simulink model "PowertrainV4"  (R2020b)
settings: Solver=VariableStepAuto  StartTime=0.0  StopTime=3000  MaxStep=0.06  RelTol=1e-3
values from neighbouring files (symbols this model uses):
  b = b +0.0001    (= 0.000245823376094)    [MotorSpecsForSimscape.m]
  F_drag = 0.5*1.2*0.089*0.42    (= 0.022428)    [MotorSpecsForSimscape.m]
  F_roll = 120 * 9.81 * 0.005    (= 5.886)    [MotorSpecsForSimscape.m]
  gearR = 46/11    (= 4.18181818182)    [MotorSpecsForSimscape.m]
  K = 0.0385    [MotorSpecsForSimscape.m]
  R = 0.103    [MotorSpecsForSimscape.m]
  Rs = 0.4    [MotorSpecsForSimscape.m]
  startup_t = 50    [MotorSpecsForSimscape.m]
  V_control = 24    [MotorSpecsForSimscape.m]
libraries: fl_lib x22, nesl_utility x11, sdl_lib x4, ee_lib x2
settings Model: Creator=Tom  LastModifiedBy=Tom
settings SolverCC: InitialStep=0.025

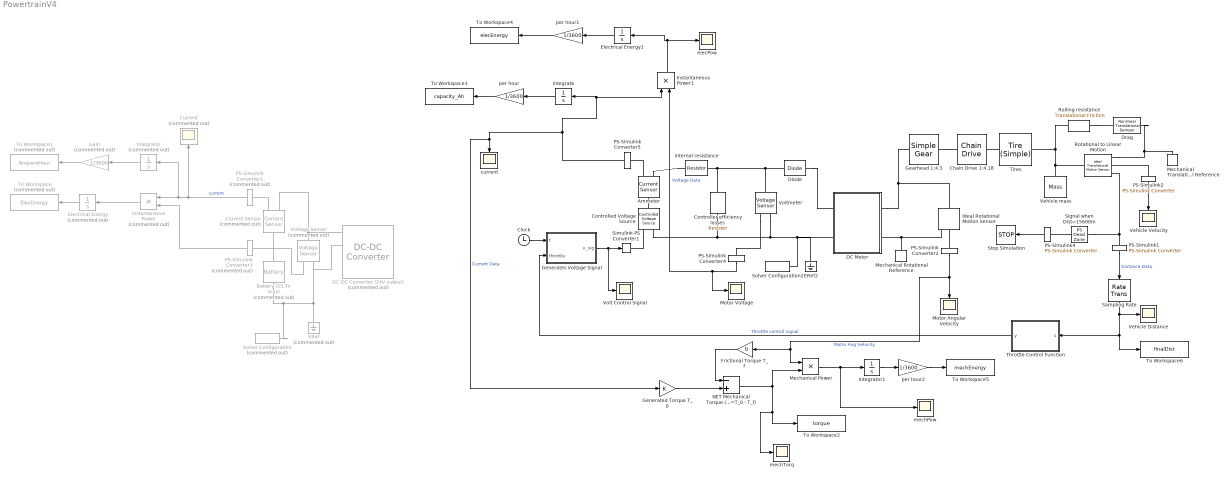
== system PowertrainV4 ==
  " Controlled Voltage Source" : fl_lib/Electrical/Electrical Sources/Controlled Voltage Source
  Ammeter : fl_lib/Electrical/Electrical Sensors/Current Sensor
  Battery (53.3V max) : ee_lib/Sources/Battery  Commented=on  Vnom=V0 V  prm_dir=1  R1_dis=2 Ohm  R1_ch=2 Ohm  R1=Rs Ohm  prm_AH=2  AH=AH0 hr*A  V1=V1 V  AH1=AH1 hr*A  prm_R2=1  R2=2000 Ohm  prm_dyn=1  Rp1=0.005 Ohm  tau1=30 s  Rp2=0.005 Ohm  tau2=30 s  Rp3=0.005 Ohm  tau3=30 s  Rp4=0.005 Ohm  tau4=30 s  Rp5=0.005 Ohm  tau5=30 s  prm_fade=1  N_fade=100  AH_fade=45 hr*A  R1_fade=2.02 Ohm  R1_ch_fade=2.02 Ohm  V1_fade=10.35 V  i_specify=off  i_priority=None  i=0 A  i_nominal_specify=off  i_nominal_unit=A  i_nominal_value=1  v_specify=off  v_priority=None  v=0 V  v_nominal_specify=off  v_nominal_unit=V  v_nominal_value=1  charge_specify=on  charge_priority=High  charge=AH0 hr*A  charge_nominal_specify=off  charge_nominal_unit=hr*A  charge_nominal_value=1  num_cycles_specify=off  num_cycles_priority=High  num_cycles=0  num_cycles_nominal_specify=off  num_cycles_nominal_unit=1  num_cycles_nominal_value=1  thermal_mass=30000 J/K  Tmeas=298.15 K  Vnom_T2=12 V  R1_T2=2.2 Ohm  R1_T2_dis=2.2 Ohm  R1_T2_ch=2.2 Ohm  V1_T2=11.4 V  R2_T2=2200 Ohm  Rp1_T2=0.005 Ohm  tau1_T2=30 s  Rp2_T2=0.005 Ohm  tau2_T2=30 s  Rp3_T2=0.005 Ohm  tau3_T2=30 s  Rp4_T2=0.005 Ohm  tau4_T2=30 s  Rp5_T2=0.005 Ohm  tau5_T2=30 s  Tmeas2=273.15 K  temperature_specify=off  temperature_priority=High  temperature=298.15 K  temperature_nominal_specify=off  temperature_nominal_unit=K  temperature_nominal_value=1
  Chain Drive 1:4.18 : sdl_lib/Couplings & Drives/Chain Drive  chain_model=sdl.enum.chain_model.ideal  radius_a=20 mm  radius_b=20*gearR mm  slack=50 mm  k_chain=1e5 N/m  mu_visc_chain=5 N/(m/s)  mu_visc_a=0 N*m/(rad/s)  mu_visc_b=0 N*m/(rad/s)  breakable=sdl.enum.max_tension.off  F_max=1e6 N  x_specify=off  x_priority=High  x=0 mm  x_nominal_specify=off  x_nominal_unit=mm  x_nominal_value=1
      settings: SourceProductBaseCode=LD  InternalSimscapePortConfiguration="{\"Bottom\":[],\"Left\":[{\"id\":\"A\",\"label\":\"A\",\"type\":\"foundation.mechanical.rotational.rotational\"}],\"Right\":[{\"id\":\"B\",\"label\":\"B\",\"type\":\"foundation.mechanical.rotational.rotational\"}],\"Top\":[]}"
  "Clock " : Clock
  Controller efficiency losses : fl_lib/Electrical/Electrical Elements/Resistor  R=30 Ohm  i_specify=off  i_priority=None  i=0 A  i_nominal_specify=off  i_nominal_unit=A  i_nominal_value=1  v_specify=off  v_priority=None  v=0 V  v_nominal_specify=off  v_nominal_unit=V  v_nominal_value=1
  Current : Scope  Commented=on
  Current Sensor : fl_lib/Electrical/Electrical Sensors/Current Sensor  Commented=on
  DC Motor : Subsystem
  "DC-DC Converter (24V output) " : ee_lib/Semiconductors & Converters/Converters/DC-DC Converter  Commented=on  Vref_option=ee.enum.converters.voltageref.external  v_ref=V_control V  P_rated=200 W  droop_param=1  droop=0.1 V/A  droop_percent=2  reversible=0  efficiency=0.9  P_fixed=1 W  model_dynamics=0  tau=0.02 s  v_ini=10 V  G_diode=1e-8 1/Ohm  i1_max=300 A  fault_condition=1  fault_threshold=0.5  thermal_mass=100 J/K  initial_temperature=298.15 K
      settings: SourceProductBaseCode=PS  InternalSimscapePortConfiguration="{\"Bottom\":[],\"Left\":[{\"id\":\"p1\",\"label\":\"1+\",\"type\":\"foundation.electrical.electrical\"},{\"id\":\"n1\",\"label\":\"1-\",\"type\":\"foundation.electrical.electrical\"},{\"id\":\"Vref\",\"label\":\"Vref\",\"type\":\"input\"},{\"id\":\"F\",\"label\":\"F\",\"type\":\"input\"}],\"Right\":[{\"id\":\"p2\",\"label\":\"2+\",\"type\":\"foundation.electrical.electrical\"},{\"id\":\"n2\",\"label\":\"2-\",\"type\":\"foundation.electrical.electrical\"}],\"Top\":[]}"
  Diode : fl_lib/Electrical/Electrical Elements/Diode  Vf=0.5 V  Ron=0.1 Ohm  Goff=0.0001 1/Ohm  i_specify=off  i_priority=None  i=0 A  i_nominal_specify=off  i_nominal_unit=A  i_nominal_value=1  v_specify=off  v_priority=None  v=0 V  v_nominal_specify=off  v_nominal_unit=V  v_nominal_value=1
  Drag : sdl_lib/Couplings & Drives/Springs & Dampers/Nonlinear Translational Damper  parameterization=1  symmetry=1  coefficient_vector=[0, F_drag, 0, 0, 0] N/(m/s)  extension_coefficient_vector=[10, 0, 1, 0, .1] N/(m/s)  contraction_coefficient_vector=[100, -1, 10, 0, 0] N/(m/s)  velocity_vector=[-1, -.5, -.3, -.1, .1, .3, .5, 1] m/s  force_vector=[-100, -40, -20, -5, 5, 20, 40, 100] N  interp_method=simscape.enum.interpolation.linear  extrap_method=simscape.enum.extrapolation.linear
      settings: SourceProductBaseCode=LD  InternalSimscapePortConfiguration="{\"Bottom\":[],\"Left\":[{\"id\":\"R\",\"label\":\"R\",\"type\":\"foundation.mechanical.translational.translational\"}],\"Right\":[{\"id\":\"C\",\"label\":\"C\",\"type\":\"foundation.mechanical.translational.translational\"}],\"Top\":[]}"
  ERef : fl_lib/Electrical/Electrical Elements/Electrical Reference  Commented=on
  ERef2 : fl_lib/Electrical/Electrical Elements/Electrical Reference
  Electrical Energy : Integrator  Commented=on
  Electrical Energy1 : Integrator
  Frictional Torque T_f : Gain  Gain=b
  Gain : Gain  Commented=on  Gain=1/3600
  Gearhead 1:4.3 : sdl_lib/Gears/Simple Gear  ratio=4.3  rotation_direction=sdl.enum.shaftOutputDirection.same  friction_model=sdl.enum.gear_efficiencies_load.constant  mu_visc=[0, 0] N*m/(rad/s)  T_noload=0.1 N*m  T_nom=5 N*m  efficiency_nom=0.8  efficiency=0.9  temperature_TLU=[280, 300, 320] K  load_TLU=[1, 5, 10] N*m  efficiency_TLU=[.95, .9, .85]  efficiency_TLU2=[.85, .8, .75; .95, .9, .85; .85, .8, .7]  w_thr=0.01 rad/s  pwr_thr=0.001 W  thermal_mass=50 J/K  enable_faults=simscape.enum.onoff.off  efficiency_fault=0.05  external_fault=simscape.enum.onoff.off  temporal_fault=simscape.enum.onoff.off  fault_time=5 s  fault_angles=pi / 12 rad  report_fault=simscape.enum.assert.action.none  temperature_specify=off  temperature_priority=High  temperature=300 K  temperature_nominal_specify=off  temperature_nominal_unit=K  temperature_nominal_value=1
  Generated Torque T_0 : Gain  Gain=K
  Generates Voltage Signal : MATLAB Function  TreatAsAtomicUnit=on
  Ideal Rotational Motion Sensor : fl_lib/Mechanical/Mechanical Sensors/Ideal Rotational Motion Sensor  wrap_angle=simscape.enum.onoff.off  offset=0 rad
  Instantaneous Power : Product  Commented=on
  Instantaneous Power1 : Product
  Integrator : Integrator  Commented=on
  Integrator1 : Integrator
  Mechanical Rotational Reference : fl_lib/Mechanical/Rotational Elements/Mechanical Rotational Reference
  Mechanical Translational Reference : fl_lib/Mechanical/Translational Elements/Mechanical Translational Reference
  Mechanical Power : Product
  Motor Angular Velocity : Scope
  "Motor Voltage " : Scope
  NET Mechanical Torque (T=T_0 - T_f) : Sum  Inputs=-+
  PS-Simulink Converter1 : nesl_utility/PS-Simulink Converter  Commented=on  PhysicalDomain=network_engine_domain  SubClassName=ps_output  LeftPortType=input  RightPortType=output  PseudoPeriodic=off  Frequencies=[]  Unit=1  AffineConversion=off
  PS-Simulink Converter2 : nesl_utility/PS-Simulink Converter  PhysicalDomain=network_engine_domain  SubClassName=ps_output  LeftPortType=input  RightPortType=output  PseudoPeriodic=off  Frequencies=[]  Unit=1  AffineConversion=off
  PS-Simulink Converter3 : nesl_utility/PS-Simulink Converter  Commented=on  PhysicalDomain=network_engine_domain  SubClassName=ps_output  LeftPortType=input  RightPortType=output  PseudoPeriodic=off  Frequencies=[]  Unit=1  AffineConversion=off
  PS-Simulink Converter4 : nesl_utility/PS-Simulink Converter  PhysicalDomain=network_engine_domain  SubClassName=ps_output  LeftPortType=input  RightPortType=output  PseudoPeriodic=off  Frequencies=[]  Unit=1  AffineConversion=off
  PS-Simulink Converter5 : nesl_utility/PS-Simulink Converter  PhysicalDomain=network_engine_domain  SubClassName=ps_output  LeftPortType=input  RightPortType=output  PseudoPeriodic=off  Frequencies=[]  Unit=1  AffineConversion=off
  PS-Simulink1 : nesl_utility/PS-Simulink Converter  PhysicalDomain=network_engine_domain  SubClassName=ps_output  LeftPortType=input  RightPortType=output  PseudoPeriodic=off  Frequencies=[]  Unit=m  AffineConversion=off
  PS-Simulink2 : nesl_utility/PS-Simulink Converter  PhysicalDomain=network_engine_domain  SubClassName=ps_output  LeftPortType=input  RightPortType=output  PseudoPeriodic=off  Frequencies=[]  Unit=m/s  AffineConversion=off
  PS-Simulink4 : nesl_utility/PS-Simulink Converter  PhysicalDomain=network_engine_domain  SubClassName=ps_output  LeftPortType=input  RightPortType=output  PseudoPeriodic=off  Frequencies=[]  Unit=m  AffineConversion=off
  Rolling resistance : fl_lib/Mechanical/Translational Elements/Translational Friction  brkwy_frc=F_roll + 0.5 N  brkwy_vel=0.01 m/s  Col_frc=F_roll N  visc_coef=0.1 N/(m/s)  v_specify=off  v_priority=None  v=0 m/s  v_nominal_specify=off  v_nominal_unit=m/s  v_nominal_value=1  f_specify=off  f_priority=None  f=0 N  f_nominal_specify=off  f_nominal_unit=N  f_nominal_value=1
      settings: SourceProductBaseCode=SS  InternalSimscapePortConfiguration="{\"Bottom\":[],\"Left\":[{\"id\":\"R\",\"label\":\"R\",\"type\":\"foundation.mechanical.translational.translational\"}],\"Right\":[{\"id\":\"C\",\"label\":\"C\",\"type\":\"foundation.mechanical.translational.translational\"}],\"Top\":[]}"
  Rotational to Linear Motion : fl_lib/Mechanical/Mechanical Sensors/Ideal Translational Motion Sensor  offset=0 m
  Sampling Rate : RateTransition  OutPortSampleTime=0.05
  Signal when Dist=15600m : fl_lib/Physical Signals/Nonlinear Operators/PS Dead Zone  upper_limit=15620 m  lower_limit=0 m
      settings: SourceProductBaseCode=SS  InternalSimscapePortConfiguration="{\"Bottom\":[],\"Left\":[{\"id\":\"I\",\"label\":\"\",\"type\":\"input\"}],\"Right\":[{\"id\":\"O\",\"label\":\"\",\"type\":\"output\"}],\"Top\":[]}"
  Simulink-PS Converter1 : nesl_utility/Simulink-PS Converter  PhysicalDomain=network_engine_domain  SubClassName=ps_input  LeftPortType=input  RightPortType=output  PseudoPeriodic=off  Frequencies=[]  NoiseDistribution=none  NoiseParameters=[]  Unit=1  AffineConversion=off  FilteringAndDerivatives=filter  SimscapeFilterOrder=1  InputFilterTimeConstant=0.001  UdotUserProvided=0
  Solver Configuration : nesl_utility/Solver Configuration  Commented=on  PhysicalDomain=network_engine_domain  SubClassName=solver  LeftPortType=input  RightPortType=generic  Tones=[]  Harmonics=[]  SimulateNoise=off  Profile=off  UseLocalSampling=off  EnableSwitchedLinearOptims=on  FrequencyDomain=off  UseCCode=off  RelTol=0.001  AbsTol=1e-06  MinStep=1e-09  ToWorkspace=off  RevertToSquareIcSolve=off  NumHomotopyIterations=100  PhasorMode=off  PhasorModeNumHarmonics=1  DoDC=off  ResidualTolerance=1e-9  UseLocalSolver=off  LocalSolverChoice=NE_BACKWARD_EULER_ADVANCER  LocalSolverSampleTime=5e-6  DoFixedCost=off  MaxNonlinIter=4  MaxModeIter=2  ComputeImpulses=off  ImpulseIterations=2  LinearAlgebra=auto  EquationFormulation=NE_TIME_EF  DelaysMemoryBudget=1024  AutomaticFiltering=on  FilteringTimeConstant=0.001  PartitionStorageMethod=AS_NEEDED  PartitionMemoryBudget=1024  PartitionMethod=FAST
  Solver Configuration2 : nesl_utility/Solver Configuration  PhysicalDomain=network_engine_domain  SubClassName=solver  LeftPortType=input  RightPortType=generic  Tones=[]  Harmonics=[]  SimulateNoise=off  Profile=off  UseLocalSampling=off  EnableSwitchedLinearOptims=on  FrequencyDomain=off  UseCCode=off  RelTol=0.001  AbsTol=1e-06  MinStep=1e-09  ToWorkspace=off  RevertToSquareIcSolve=off  NumHomotopyIterations=100  PhasorMode=off  PhasorModeNumHarmonics=1  DoDC=off  ResidualTolerance=1e-9  UseLocalSolver=off  LocalSolverChoice=NE_BACKWARD_EULER_ADVANCER  LocalSolverSampleTime=5e-6  DoFixedCost=off  MaxNonlinIter=4  MaxModeIter=2  ComputeImpulses=off  ImpulseIterations=2  LinearAlgebra=auto  EquationFormulation=NE_TIME_EF  DelaysMemoryBudget=1024  AutomaticFiltering=on  FilteringTimeConstant=0.001  PartitionStorageMethod=AS_NEEDED  PartitionMemoryBudget=1024  PartitionMethod=FAST
  Stop Simulation : Stop
  Throttle Control Function : MATLAB Function  TreatAsAtomicUnit=on
  Tires : sdl_lib/Tires & Vehicles/Tire (Simple)  r_tire=0.254 m  model_compliance=0  stiffness=1e6 N/m  damping=1000 N/(m/s)  model_inertia=1  tire_inertia=0.5 kg*m^2  initial_velocity=0 rad/s
      settings: SourceProductBaseCode=LD  InternalSimscapePortConfiguration="{\"Bottom\":[],\"Left\":[{\"id\":\"A\",\"label\":\"A\",\"type\":\"foundation.mechanical.rotational.rotational\"}],\"Right\":[{\"id\":\"H\",\"label\":\"H\",\"type\":\"foundation.mechanical.translational.translational\"}],\"Top\":[]}"
  To Workspace : ToWorkspace  Commented=on  VariableName=ElecEnergy  SaveFormat=Timeseries  SampleTime=-1
      settings: MaxDataPoints=1
  To Workspace1 : ToWorkspace  Commented=on  VariableName=AmpereHour  SaveFormat=Timeseries  SampleTime=-1
      settings: MaxDataPoints=1
  To Workspace2 : ToWorkspace  VariableName=torque  SaveFormat=Timeseries  SampleTime=0.2
  To Workspace3 : ToWorkspace  VariableName=capacity_Ah  SaveFormat=Timeseries  SampleTime=-1
      settings: MaxDataPoints=1
  To Workspace4 : ToWorkspace  VariableName=elecEnergy  SaveFormat=Timeseries  SampleTime=-1
      settings: MaxDataPoints=1
  To Workspace5 : ToWorkspace  VariableName=mechEnergy  SaveFormat=Timeseries  SampleTime=-1
      settings: MaxDataPoints=1
  To Workspace6 : ToWorkspace  VariableName=finalDist  SaveFormat=Timeseries  SampleTime=-1
      settings: MaxDataPoints=1
  Vehicle Distance : Scope
  Vehicle Velocity : Scope
  Vehicle mass : fl_lib/Mechanical/Translational Elements/Mass  mass=M kg  num_ports=foundation.enum.numPorts2.one  v_specify=off  v_priority=High  v=0 m/s  v_nominal_specify=off  v_nominal_unit=m/s  v_nominal_value=1  f_specify=off  f_priority=None  f=0 N  f_nominal_specify=off  f_nominal_unit=N  f_nominal_value=1
  Volt Control Signal : Scope
  Voltage Sensor : fl_lib/Electrical/Electrical Sensors/Voltage Sensor  Commented=on
  Voltmeter : fl_lib/Electrical/Electrical Sensors/Voltage Sensor
  current : Scope
  elecPow : Scope
  integrate : Integrator
  internal resistance : fl_lib/Electrical/Electrical Elements/Resistor  R=Rs Ohm  i_specify=off  i_priority=None  i=0 A  i_nominal_specify=off  i_nominal_unit=A  i_nominal_value=1  v_specify=off  v_priority=None  v=0 V  v_nominal_specify=off  v_nominal_unit=V  v_nominal_value=1
  mechPow : Scope
  mechTorq : Scope
  per hour : Gain  Gain=1/3600
  per hour1 : Gain  Gain=1/3600
  per hour2 : Gain  Gain=1/3600
  wires:
  PS-Simulink Converter2/1 -> Motor Angular Velocity/1, Mechanical Power/1, Frictional Torque T_f/1  "Motor Ang Velocity"
  Throttle Control Function/1(y) -> Generates Voltage Signal/2(throttle)  "Throttle control signal"
  PS-Simulink4/1 -> Stop Simulation/1
  PS-Simulink2/1 -> Vehicle Velocity/1
  PS-Simulink1/1 -> Sampling Rate/1  "Distance Data"
  Sampling Rate/1 -> Vehicle Distance/1, To Workspace6/1, Throttle Control Function/1(s)
  Electrical Energy/1 -> To Workspace/1
  PS-Simulink Converter1/1 -> Current/1, Integrator/1, Instantaneous Power/1  "current"
  PS-Simulink Converter3/1 -> Instantaneous Power/2
  Instantaneous Power/1 -> Electrical Energy/1
  Integrator/1 -> Gain/1
  Gain/1 -> To Workspace1/1
  Mechanical Power/1 -> mechPow/1, Integrator1/1
  NET Mechanical Torque (T=T_0 - T_f)/1 -> Mechanical Power/2, mechTorq/1, To Workspace2/1
  Frictional Torque T_f/1 -> NET Mechanical Torque (T=T_0 - T_f)/1
  PS-Simulink Converter4/1 -> Instantaneous Power1/2, "Motor Voltage "/1  "Voltage Data"
  Generated Torque T_0/1 -> NET Mechanical Torque (T=T_0 - T_f)/2
  "Clock "/1 -> Generates Voltage Signal/1(t)
  Generates Voltage Signal/1(v_sig) -> Volt Control Signal/1, Simulink-PS Converter1/1
  PS-Simulink Converter5/1 -> Instantaneous Power1/1, integrate/1, current/1, Generated Torque T_0/1  "Current Data"
  integrate/1 -> per hour/1
  per hour/1 -> To Workspace3/1
  Electrical Energy1/1 -> per hour1/1
  Instantaneous Power1/1 -> Electrical Energy1/1, elecPow/1
  Integrator1/1 -> per hour2/1
  per hour1/1 -> To Workspace4/1
  per hour2/1 -> To Workspace5/1
  connections:
  Rotational to Linear Motion/LConn1 -- Vehicle mass/LConn1 -- Tires/RConn1 -- Rolling resistance/LConn1
  Ideal Rotational Motion Sensor/RConn1 -- Mechanical Rotational Reference/LConn1 -- DC Motor/RConn2
  Rotational to Linear Motion/RConn1 -- Drag/RConn1 -- Mechanical Translational Reference/LConn1
  Signal when Dist=15600m/LConn1 -- PS-Simulink1/LConn1 -- Rotational to Linear Motion/RConn3
  DC Motor/RConn1 -- Ideal Rotational Motion Sensor/LConn1 -- Gearhead 1:4.3/LConn1
  Signal when Dist=15600m/RConn1 -- PS-Simulink4/LConn1
  Tires/LConn1 -- Chain Drive 1:4.18/RConn1
  PS-Simulink Converter2/LConn1 -- Ideal Rotational Motion Sensor/RConn2
  PS-Simulink2/LConn1 -- Rotational to Linear Motion/RConn2
  Gearhead 1:4.3/RConn1 -- Chain Drive 1:4.18/LConn1
  Solver Configuration/RConn1 -- Voltage Sensor/RConn2 -- "DC-DC Converter (24V output) "/LConn2 -- ERef/LConn1 -- Battery (53.3V max)/RConn1
  Current Sensor/LConn1 -- Battery (53.3V max)/LConn1
  Voltage Sensor/LConn1 -- Current Sensor/RConn2 -- "DC-DC Converter (24V output) "/LConn1
  Current Sensor/RConn1 -- PS-Simulink Converter1/LConn1
  Voltage Sensor/RConn1 -- PS-Simulink Converter3/LConn1
  Rolling resistance/RConn1 -- Drag/LConn1
  " Controlled Voltage Source"/RConn1 -- Simulink-PS Converter1/RConn1
  Voltmeter/RConn1 -- PS-Simulink Converter4/LConn1
  Ammeter/RConn1 -- PS-Simulink Converter5/LConn1
  " Controlled Voltage Source"/LConn1 -- Ammeter/LConn1
  " Controlled Voltage Source"/RConn2 -- ERef2/LConn1 -- DC Motor/LConn2 -- Solver Configuration2/RConn1 -- Voltmeter/RConn2 -- Controller efficiency losses/RConn1
  internal resistance/RConn1 -- Diode/LConn1 -- Voltmeter/LConn1 -- Controller efficiency losses/LConn1
  internal resistance/LConn1 -- Ammeter/RConn2
  Diode/RConn1 -- DC Motor/LConn1

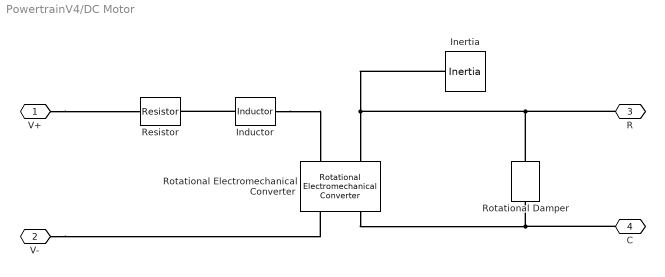
== system PowertrainV4/DC Motor ==
  Inductor : fl_lib/Electrical/Electrical Elements/Inductor  l=L H  r=0 Ohm  g=1e-9 1/Ohm  i_specify=off  i_priority=None  i=0 A  i_nominal_specify=off  i_nominal_unit=A  i_nominal_value=1  v_specify=off  v_priority=None  v=0 V  v_nominal_specify=off  v_nominal_unit=V  v_nominal_value=1  i_L_specify=off  i_L_priority=High  i_L=0 A  i_L_nominal_specify=off  i_L_nominal_unit=A  i_L_nominal_value=1
  Inertia : fl_lib/Mechanical/Rotational Elements/Inertia  inertia=J kg*m^2  num_ports=foundation.enum.numPorts2.one  w_specify=off  w_priority=High  w=0 rad/s  w_nominal_specify=off  w_nominal_unit=rad/s  w_nominal_value=1  t_specify=off  t_priority=None  t=0 N*m  t_nominal_specify=off  t_nominal_unit=N*m  t_nominal_value=1
  Resistor : fl_lib/Electrical/Electrical Elements/Resistor  R=R Ohm  i_specify=off  i_priority=None  i=0 A  i_nominal_specify=off  i_nominal_unit=A  i_nominal_value=1  v_specify=off  v_priority=None  v=0 V  v_nominal_specify=off  v_nominal_unit=V  v_nominal_value=1
  Rotational Electromechanical Converter : fl_lib/Electrical/Electrical Elements/Rotational Electromechanical Converter  K=K V/(rad/s)  i_specify=off  i_priority=None  i=0 A  i_nominal_specify=off  i_nominal_unit=A  i_nominal_value=1  v_specify=off  v_priority=None  v=0 V  v_nominal_specify=off  v_nominal_unit=V  v_nominal_value=1  t_specify=off  t_priority=None  t=0 N*m  t_nominal_specify=off  t_nominal_unit=N*m  t_nominal_value=1  w_specify=off  w_priority=None  w=0 rad/s  w_nominal_specify=off  w_nominal_unit=rad/s  w_nominal_value=1
  Rotational Damper : fl_lib/Mechanical/Rotational Elements/Rotational Damper  D=b N*m/(rad/s)  w_specify=off  w_priority=None  w=0 rad/s  w_nominal_specify=off  w_nominal_unit=rad/s  w_nominal_value=1  t_specify=off  t_priority=None  t=0 N*m  t_nominal_specify=off  t_nominal_unit=N*m  t_nominal_value=1
  V+ : PMIOPort  Side=Left
  V- : PMIOPort  Port=2  Side=Left
  R : PMIOPort  Port=3  Side=Right
  C : PMIOPort  Port=4  Side=Right
  connections:
  Inertia/LConn1 -- R/RConn1 -- Rotational Damper/RConn1 -- Rotational Electromechanical Converter/LConn2
  V+/RConn1 -- Resistor/LConn1
  Inductor/LConn1 -- Resistor/RConn1
  Inductor/RConn1 -- Rotational Electromechanical Converter/LConn1
  Rotational Electromechanical Converter/RConn2 -- C/RConn1 -- Rotational Damper/LConn1
  V-/RConn1 -- Rotational Electromechanical Converter/RConn1

== matlab function PowertrainV4/Generates Voltage Signal ==
  data: t input; throttle input; v_sig output; V_control parameter; startup_t parameter
function v_sig = fcn(t, throttle, V_control, startup_t) 
%note - V_control has been set to a parameter in 'Edit data' which is why
%it does not appear as an input port on Simulink

%create the start ramp input, then hold signal at V_control = 24V
if t <= startup_t
    v_sig = (1/startup_t)*t*V_control;
else
    v_sig = V_control;
    %account for throttle signal
    if (throttle == 0)
        v_sig = 0.5*V_control; %half power
    end
end

end

== matlab function PowertrainV4/Throttle Control Function ==
  data: s input; y output; a parameter
function y = lap_progress(s, a)
%array 'a' contains 142 data points per lap, indicating 1 = on and 0 = off.

%relate distance progression to corresponding element in array 'a':
prog = floor(s/15600 * 142*13) +1; % floor rounds down, so +1 to round up

if (prog <= 0)
    prog = 1;
end

if (prog <= 142) %Lap 1
    y = a(prog, 1); %column 1 contains 1st lap data

elseif (142 < prog) && (prog <= 142*12) %Laps 2 -> 12
    
    lap_num = floor(prog/142)+ 1; %find the lap number
    ind = prog - 142*(lap_num-1); %find index of column 2
    if (ind <= 0)
        ind = 1; 
    end

    y = a(ind, 2); %output

else %Lap 13 (final)
    ind = prog-142*12; %find index for final lap
    if (ind > 142)
        ind = 142;
    end

    y = a(ind, 3); %output
end     

end
